simulink model "to_del"  (R2020b)
settings: Solver=VariableStepAuto  StartTime=0.0  StopTime=10.0  RelTol=1e-3
values from neighbouring files (symbols this model uses):
  w = 0.03    [cost_function.m]    (also in main.m = file.load_oc_without_noise(2,:); testttttt.m = 0.5)
libraries: fuzblock x1
settings Model: Creator=maloc  LastModifiedBy=maloc

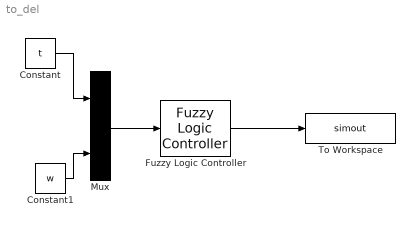
== system to_del ==
  Constant : Constant  Value=t
  Constant1 : Constant  Value=w
  Fuzzy Logic Controller : fuzblock/Fuzzy Logic  Controller  FIS=fisi  OutputSampleNumber=2  DataType=double  FuzzifiedInputs=off  RuleFiringStrengths=off  RuleOutputs=off  AggregatedOutputs=off  SimulateUsing=Code generation  OutOfRangeInputValueMessage=warning  NoRuleFiredMessage=warning  EmptyOutputFuzzySetMessage=warning
  Mux : Mux  Inputs=2
  To Workspace : ToWorkspace  VariableName=simout  SaveFormat=Timeseries  SampleTime=-1
  wires:
  Mux/1 -> Fuzzy Logic Controller/1
  Constant/1 -> Mux/1
  Constant1/1 -> Mux/2
  Fuzzy Logic Controller/1 -> To Workspace/1
